simulink library "PrintErrorToTerminal"  (R2016b)
settings: Solver=VariableStepAuto  StartTime=0.0  StopTime=10.0  RelTol=1e-3
settings Model: Creator=MARCH  LastModifiedBy=MARCH

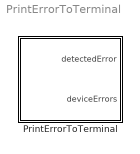
== system PrintErrorToTerminal ==
  PrintErrorToTerminal : Subsystem

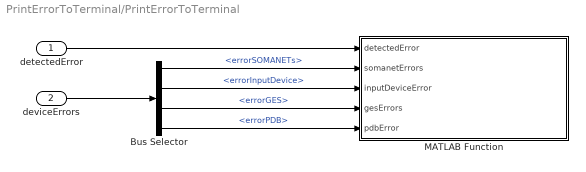
== system PrintErrorToTerminal/PrintErrorToTerminal ==
  detectedError : Inport
  deviceErrors : Inport  Port=2
  Bus Selector : BusSelector  OutputSignals=errorSOMANETs,errorInputDevice,errorGES,errorPDB
  MATLAB Function : MATLAB Function  TreatAsAtomicUnit=on
  wires:
  detectedError/1 -> MATLAB Function/1(detectedError)
  deviceErrors/1 -> Bus Selector/1
  Bus Selector/4 -> MATLAB Function/5(pdbError)  "<errorPDB>"
  Bus Selector/3 -> MATLAB Function/4(gesErrors)  "<errorGES>"
  Bus Selector/2 -> MATLAB Function/3(inputDeviceError)  "<errorInputDevice>"
  Bus Selector/1 -> MATLAB Function/2(somanetErrors)  "<errorSOMANETs>"

== matlab function PrintErrorToTerminal/MATLAB Function ==
  data: detectedError input; somanetErrors input; inputDeviceError input; gesErrors input; pdbError input
function printErrorToTerminal(detectedError, somanetErrors, inputDeviceError, gesErrors, pdbError)
% wrapper for printErrorToTerminal
printErrorToTerminal(detectedError, somanetErrors, inputDeviceError, gesErrors, pdbError);
end
